simulink model "UUV_animation"  (Simulink 8.3)
settings: Solver=ode45  StartTime=0.0  StopTime=100  RelTol=1e-3
undefined symbols (not defined in the file or in its folder): drawUUV
settings Model: Creator=beard  LastModifiedBy=jhl48
settings OptimizationCC: ExpressionDepthLimit=2147483647  InitFltsAndDblsToZero=on
settings DebuggingCC: FcnCallInpInsideContextMsg=UseLocalSettings

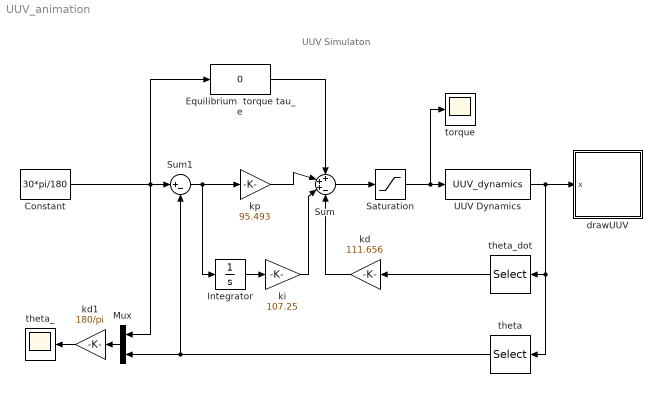
== system UUV_animation ==
  note: UUV Simulaton
  Constant : Constant  Value=30*pi/180
  Equilibrium  torque tau_e : Fcn  Expr=0
  Integrator : Integrator
  Mux : Mux  Inputs=2
  Saturation : Saturate  UpperLimit=50  LowerLimit=-50
  Sum : Sum  Inputs=+++-
  Sum1 : Sum  Inputs=|+-
  UUV Dynamics : S-Function  FunctionName=UUV_dynamics  Parameters=P  EnableBusSupport=off
  drawUUV : Subsystem
      mask init:
      | % drawing parameters
      | L = 1;
      | w = 0.3;
      | 
      | MajorAxis = 10;
      | MinorAxis = 6;
      | C_M = [0;-4];
      mask Display: image(imread('tv.jpg'))
  kd : Gain  Gain=111.656
  kd1 : Gain  Gain=180/pi
  ki : Gain  Gain=107.25
  kp : Gain  Gain=95.493
  theta : Selector  InputPortWidth=2  Indices=[1]
  theta_ : Scope
      settings: TimeRange=100  YMin=0  YMax=2250
  theta_dot : Selector  InputPortWidth=2  Indices=[2]
  torque : Scope
      settings: TimeRange=1000  YMin=-20  YMax=50
  wires:
  UUV Dynamics/1 -> drawUUV/1(x), theta/1, theta_dot/1
  Saturation/1 -> UUV Dynamics/1, torque/1
  Sum/1 -> Saturation/1
  Sum1/1 -> Integrator/1, kp/1
  Constant/1 -> Sum1/1, Equilibrium  torque tau_e/1, Mux/1
  theta_dot/1 -> kd/1
  theta/1 -> Sum1/2, Mux/2
  kd/1 -> Sum/4
  Equilibrium  torque tau_e/1 -> Sum/1
  Mux/1 -> kd1/1
  kd1/1 -> theta_/1
  kp/1 -> Sum/2
  Integrator/1 -> ki/1
  ki/1 -> Sum/3

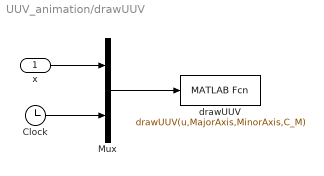
== system UUV_animation/drawUUV ==
  x : Inport
  Clock : Clock
  Mux : Mux  Inputs=2
  "drawUUV " : MATLABFcn  MATLABFcn=drawUUV(u,MajorAxis,MinorAxis,C_M)  OutputDimensions=0  SampleTime=0.1
  wires:
  Mux/1 -> "drawUUV "/1
  x/1 -> Mux/1
  Clock/1 -> Mux/2
